simulink model "ass4"  (R2018a)
settings: Solver=VariableStepAuto  StartTime=0.0  StopTime=10.0  RelTol=1e-3
settings Model: Creator=22121100  LastModifiedBy=22121100

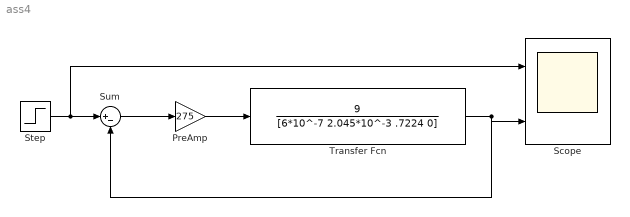
== system ass4 ==
  PreAmp : Gain  Gain=275
  Scope : Scope  NumInputPorts=2
  Step : Step  SampleTime=0
  Sum : Sum  Inputs=|+-
  Transfer Fcn : TransferFcn  Numerator=[9]  Denominator=[6*10^-7 2.045*10^-3 .7224 0]
  wires:
  Step/1 -> Scope/1, Sum/1
  Sum/1 -> PreAmp/1
  PreAmp/1 -> Transfer Fcn/1
  Transfer Fcn/1 -> Sum/2, Scope/2
